simulink model "x1_5"  (R2021a)
settings: Solver=VariableStepAuto  StartTime=0.0  StopTime=10.0  RelTol=1e-3
settings Model: Creator=Fatiha  LastModifiedBy=Fatiha

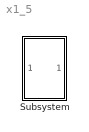
== system x1_5 ==
  Subsystem : Subsystem

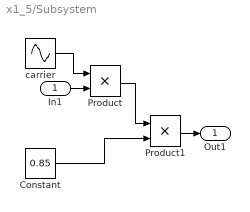
== system x1_5/Subsystem ==
  In1 : Inport
  Constant : Constant  Value=0.85
  Product : Product
  Product1 : Product
  carrier : Sin  Frequency=2*pi*500  Phase=pi/2  SampleTime=0.00001
  Out1 : Outport
  wires:
  Constant/1 -> Product1/2
  Product/1 -> Product1/1
  carrier/1 -> Product/1
  Product1/1 -> Out1/1
  In1/1 -> Product/2
